simulink model "model6_threestate_rwp"  (R2017a)
settings: Solver=ode1  StartTime=0.0  StopTime=1000  FixedStep=0.005  RelTol=1e-3  EnableMultiTasking=on
libraries: c6xlib x2, fricblocks x1
Description:
  | Real-Time Van der Pol Simulation
  | 
  | This demonstration shows a real-time version of the Simulink(R) Van der Pol
  | simulation demo. This model does not need any external signals, so it does
  | not need any data acquisition hardware or driver. This makes the model ideal
  | for first experiments with Real-Time Windows Target(TM), without need to
  | worry about proper I/O hardware configuration.
  | 
  | How to run this demo:
  | 
  |   1. Build the model using Tools -> Real-Time Workshop -> Build Model.
  |   2. Connect to the real-time code using Simulation -> Connect to target.
  |   3. Start the real-time execution using Simulation -> Start real-time code.
settings Model: SimulationMode=external  ExtModeTrigDuration=50000  Creator=Houska  LastModifiedBy=vjdixit2
settings DataIOCC: LimitDataPoints=on  SaveFormat=Array  SignalLoggingSaveFormat=ModelDataLogs  SignalLoggingName=logsOut
settings OptimizationCC: ExpressionDepthLimit=2147483647  InitFltsAndDblsToZero=on  EfficientMapNaN2IntZero=off
settings DebuggingCC: UnderspecifiedInitializationDetection=Classic  MergeDetectMultiDrivingBlocksExec=none  SignalResolutionControl=TryResolveAllWithWarning  FcnCallInpInsideContextMsg=warning  StateNameClashWarn=warning  SFUnexpectedBacktrackingDiag=warning  SFNoUnconditionalDefaultTransitionDiag=warning  SFExecutionAtInitializationDiag=none
settings ModelReferenceCC: PropagateSignalLabelsOutOfModel=off
settings RTWCC: SystemTargetFile=sldrt.tlc  TemplateMakefile=sldrt.tmf  Description=Simulink Desktop Real-Time  RTWCompilerOptimization=on
settings CodeAppCC: MaxIdLength=95
settings SimulinkDesktopRealTimeCC: TargetPreCompLibLocation=C:\MATLABR2017a\toolbox\sldrt\lib\win64  TargetLangStandard=C89/C90 (ANSI)  SupportVariableSizeSignals=off
settings ConfigComp: CovMetricSettings=dw  CovHtmlReporting=on  CovSaveCumulativeToWorkspaceVar=on  CovSaveSingleToWorkspaceVar=on  CovExternalEMLEnable=off  CovSFcnEnable=off

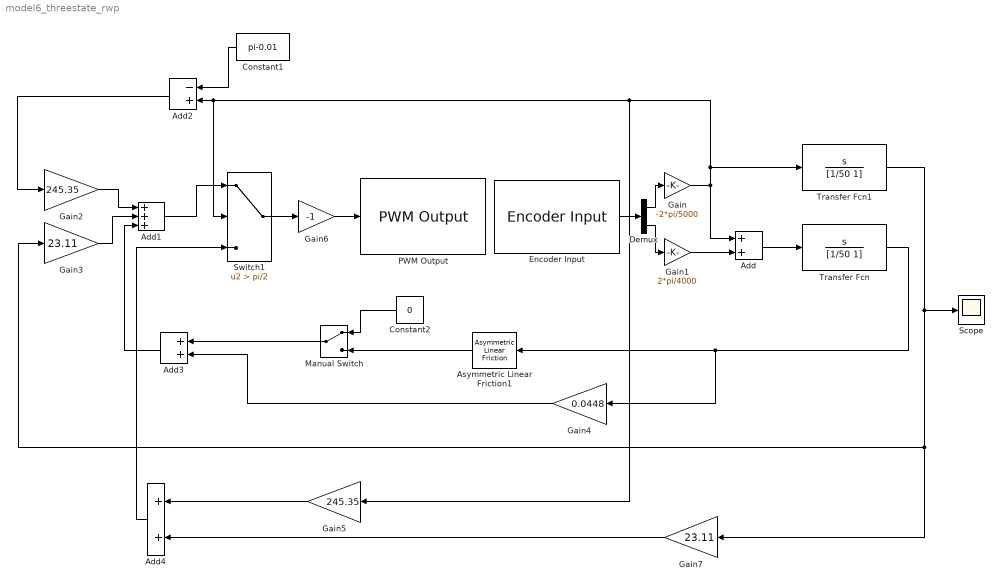
== system model6_threestate_rwp ==
  Add : Sum
  Add1 : Sum  Inputs=+++
  Add2 : Sum  Inputs=-+
  Add3 : Sum
  Add4 : Sum
  Asymmetric Linear Friction1 : fricblocks/Asymmetric  Linear Friction  intercept1=0.605*(2/3)  intercept2=-.67*(2/3)  slope1=0.0126*(2/3)  slope2=0.0128*(2/3)
  Constant1 : Constant  Value=pi-0.01
  Constant2 : Constant  Value=0
  Demux : Demux  Outputs=2
  Encoder Input : c6xlib/Encoder Input  baseAddr=0x378  channels=[0 1]  sampleTime=str2num(get_param(bdroot, 'FixedStep'))
  Gain : Gain  Gain=-2*pi/5000
  Gain1 : Gain  Gain=2*pi/4000
  Gain2 : Gain  Gain=245.35
  Gain3 : Gain  Gain=23.11
  Gain4 : Gain  Gain=0.0448
  Gain5 : Gain  Gain=245.35
  Gain6 : Gain  Gain=-1
  Gain7 : Gain  Gain=23.11
  Manual Switch : ManualSwitch
  PWM Output : c6xlib/PWM Output  baseAddr=0x378  channels=0  initialOutputs=0  finalOutputs=0  sampleTime=str2num(get_param(bdroot, 'FixedStep'))
  Scope : Scope
  Switch1 : Switch  Criteria=u2 > Threshold  Threshold=pi/2
  Transfer Fcn : TransferFcn  Numerator=[1 0]  Denominator=[1/50 1]
  Transfer Fcn1 : TransferFcn  Numerator=[1 0]  Denominator=[1/50 1]
  wires:
  Encoder Input/1 -> Demux/1
  Gain1/1 -> Add/2
  Demux/2 -> Gain1/1
  Demux/1 -> Gain/1
  Add/1 -> Transfer Fcn/1
  Gain3/1 -> Add1/2
  Gain2/1 -> Add1/1
  Add2/1 -> Gain2/1
  Add3/1 -> Add1/3
  Gain4/1 -> Add3/2
  Transfer Fcn1/1 -> Gain7/1, Gain3/1, Scope/1
  Manual Switch/1 -> Add3/1
  Asymmetric Linear Friction1/1 -> Manual Switch/2
  Constant2/1 -> Manual Switch/1
  Gain6/1 -> PWM Output/1
  Constant1/1 -> Add2/1
  Gain/1 -> Gain5/1, Switch1/2, Add2/2, Transfer Fcn1/1, Add/1
  Switch1/1 -> Gain6/1
  Add1/1 -> Switch1/1
  Gain5/1 -> Add4/1
  Gain7/1 -> Add4/2
  Transfer Fcn/1 -> Asymmetric Linear Friction1/1, Gain4/1
  Add4/1 -> Switch1/3
